simulink model "measurements"  (Simulink 8.5)
settings: Solver=ode45  StartTime=0.0  StopTime=10.0  RelTol=1e-3
libraries: powerlib x18
settings Model: Creator=Dr. Lotfifard  LastModifiedBy=PC  ExtModeTrigMode=oneshot  ExtModeArmWhenConnect=off
settings DataIOCC: LimitDataPoints=off
settings OptimizationCC: BlockReduction=off  BooleanDataType=off
settings DebuggingCC: SaveWithParameterizedLinksMsg=none  SignalResolutionControl=TryResolveAllWithWarning  MultiTaskDSMMsg=warning  MultiTaskCondExecSysMsg=none  FcnCallInpInsideContextMsg=UseLocalSettings  StrictBusMsg=None
settings HardwareCC: TargetUnknown=on

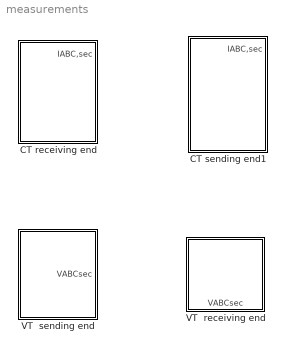
== system measurements ==
  CT receiving end : Subsystem  mask{TC=1.2}
      mask prompts: TC "Maximum Normal Current"
  CT sending end1 : Subsystem  mask{TC=1.2}
      mask prompts: TC "Maximum Normal Current"
  VT  receiving end : Subsystem  mask{TP=1000}
      mask prompts: TP "Nominal Voltage,rms"
  VT  sending end : Subsystem  mask{TP=1000}
      mask prompts: TP "Nominal Voltage,rms"

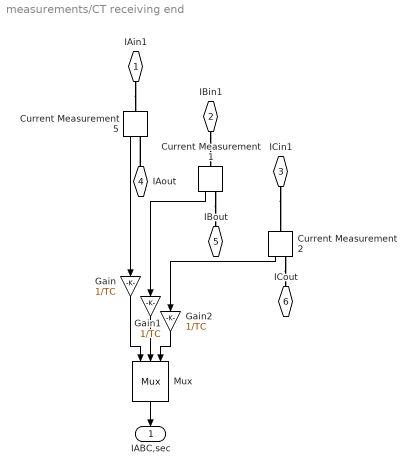
== system measurements/CT receiving end ==
  Current Measurement1 : powerlib/Measurements/Current Measurement  PhasorSimulation=off  OutputType=Complex  PSBequivalent=0
  Current Measurement2 : powerlib/Measurements/Current Measurement  PhasorSimulation=off  OutputType=Complex  PSBequivalent=0
  Current Measurement5 : powerlib/Measurements/Current Measurement  PhasorSimulation=off  OutputType=Complex  PSBequivalent=0
  Gain : Gain  Gain=1/TC  SaturateOnIntegerOverflow=on  OutDataTypeStr=Inherit: Same as input  ParamDataTypeStr=Inherit: Same as input
  Gain1 : Gain  Gain=1/TC  SaturateOnIntegerOverflow=on  OutDataTypeStr=Inherit: Same as input  ParamDataTypeStr=Inherit: Same as input
  Gain2 : Gain  Gain=1/TC  SaturateOnIntegerOverflow=on  OutDataTypeStr=Inherit: Same as input  ParamDataTypeStr=Inherit: Same as input
  Mux : Mux  Inputs=3
  IAin1 : PMIOPort  Port=1  Side=Left
  IBin1 : PMIOPort  Port=2  Side=Left
  ICin1 : PMIOPort  Port=3  Side=Left
  IAout : PMIOPort  Port=4  Side=Right
  IBout : PMIOPort  Port=5  Side=Right
  ICout : PMIOPort  Port=6  Side=Right
  IABC,sec : Outport  InitialOutput=0
  wires:
  Mux/1 -> IABC,sec/1
  Current Measurement2/1 -> Gain2/1
  Gain/1 -> Mux/1
  Gain1/1 -> Mux/2
  Gain2/1 -> Mux/3
  Current Measurement1/1 -> Gain1/1
  Current Measurement5/1 -> Gain/1
  connections:
  IAin1/RConn1 -- Current Measurement5/LConn1
  ICin1/RConn1 -- Current Measurement2/LConn1
  IBin1/RConn1 -- Current Measurement1/LConn1
  IAout/RConn1 -- Current Measurement5/RConn1
  Current Measurement1/RConn1 -- IBout/RConn1
  Current Measurement2/RConn1 -- ICout/RConn1

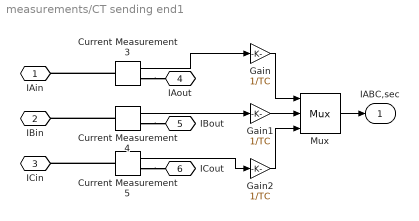
== system measurements/CT sending end1 ==
  Current Measurement3 : powerlib/Measurements/Current Measurement  PhasorSimulation=off  OutputType=Complex  PSBequivalent=0
  Current Measurement4 : powerlib/Measurements/Current Measurement  PhasorSimulation=off  OutputType=Complex  PSBequivalent=0
  Current Measurement5 : powerlib/Measurements/Current Measurement  PhasorSimulation=off  OutputType=Complex  PSBequivalent=0
  Gain : Gain  Gain=1/TC  SaturateOnIntegerOverflow=on  OutDataTypeStr=Inherit: Same as input  ParamDataTypeStr=Inherit: Same as input
  Gain1 : Gain  Gain=1/TC  SaturateOnIntegerOverflow=on  OutDataTypeStr=Inherit: Same as input  ParamDataTypeStr=Inherit: Same as input
  Gain2 : Gain  Gain=1/TC  SaturateOnIntegerOverflow=on  OutDataTypeStr=Inherit: Same as input  ParamDataTypeStr=Inherit: Same as input
  Mux : Mux  Inputs=3
  IAin : PMIOPort  Port=1  Side=Left
  IBin : PMIOPort  Port=2  Side=Left
  ICin : PMIOPort  Port=3  Side=Left
  IAout : PMIOPort  Port=4  Side=Right
  IBout : PMIOPort  Port=5  Side=Right
  ICout : PMIOPort  Port=6  Side=Right
  IABC,sec : Outport  InitialOutput=0
  wires:
  Mux/1 -> IABC,sec/1
  Gain/1 -> Mux/1
  Gain1/1 -> Mux/2
  Gain2/1 -> Mux/3
  Current Measurement3/1 -> Gain/1
  Current Measurement4/1 -> Gain1/1
  Current Measurement5/1 -> Gain2/1
  connections:
  Current Measurement4/RConn1 -- IBout/RConn1
  Current Measurement3/LConn1 -- IAin/RConn1
  Current Measurement4/LConn1 -- IBin/RConn1
  Current Measurement3/RConn1 -- IAout/RConn1
  Current Measurement5/LConn1 -- ICin/RConn1
  Current Measurement5/RConn1 -- ICout/RConn1

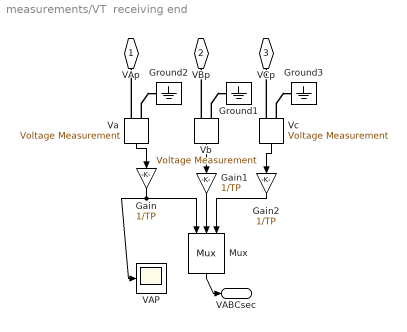
== system measurements/VT  receiving end ==
  Gain : Gain  Gain=1/TP  SaturateOnIntegerOverflow=on  OutDataTypeStr=Inherit: Same as input  ParamDataTypeStr=Inherit: Same as input
  Gain1 : Gain  Gain=1/TP  SaturateOnIntegerOverflow=on  OutDataTypeStr=Inherit: Same as input  ParamDataTypeStr=Inherit: Same as input
  Gain2 : Gain  Gain=1/TP  SaturateOnIntegerOverflow=on  OutDataTypeStr=Inherit: Same as input  ParamDataTypeStr=Inherit: Same as input
  Ground1 : powerlib/Elements/Ground  LConnTagsString=a
  Ground2 : powerlib/Elements/Ground  LConnTagsString=a
  Ground3 : powerlib/Elements/Ground  LConnTagsString=a
  Mux : Mux  Inputs=3
  VAP : Scope
      settings: TickLabels=on  YMin=-1.5  YMax=1.75
  Va : powerlib/Measurements/Voltage Measurement  PhasorSimulation=off  OutputType=Complex  PSBequivalent=0
  Vb : powerlib/Measurements/Voltage Measurement  PhasorSimulation=off  OutputType=Complex  PSBequivalent=0
  Vc : powerlib/Measurements/Voltage Measurement  PhasorSimulation=off  OutputType=Complex  PSBequivalent=0
  VAp : PMIOPort  Port=1  Side=Left
  VBp : PMIOPort  Port=2  Side=Left
  VCp : PMIOPort  Port=3  Side=Left
  VABCsec : Outport
  wires:
  Gain/1 -> VAP/1, Mux/1
  Mux/1 -> VABCsec/1
  Gain2/1 -> Mux/3
  Gain1/1 -> Mux/2
  Vb/1 -> Gain1/1
  Vc/1 -> Gain2/1
  Va/1 -> Gain/1
  connections:
  Va/LConn1 -- VAp/RConn1
  Va/LConn2 -- Ground2/LConn1
  Vb/LConn1 -- VBp/RConn1
  Vb/LConn2 -- Ground1/LConn1
  Vc/LConn1 -- VCp/RConn1
  Vc/LConn2 -- Ground3/LConn1

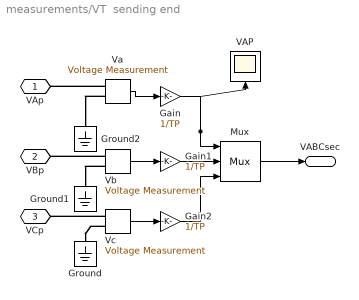
== system measurements/VT  sending end ==
  Gain : Gain  Gain=1/TP  SaturateOnIntegerOverflow=on  OutDataTypeStr=Inherit: Same as input  ParamDataTypeStr=Inherit: Same as input
  Gain1 : Gain  Gain=1/TP  SaturateOnIntegerOverflow=on  OutDataTypeStr=Inherit: Same as input  ParamDataTypeStr=Inherit: Same as input
  Gain2 : Gain  Gain=1/TP  SaturateOnIntegerOverflow=on  OutDataTypeStr=Inherit: Same as input  ParamDataTypeStr=Inherit: Same as input
  Ground : powerlib/Elements/Ground  LConnTagsString=a
  Ground1 : powerlib/Elements/Ground  LConnTagsString=a
  Ground2 : powerlib/Elements/Ground  LConnTagsString=a
  Mux : Mux  Inputs=3
  VAP : Scope
      settings: TickLabels=on  YMin=-1.5  YMax=1.75
  Va : powerlib/Measurements/Voltage Measurement  PhasorSimulation=off  OutputType=Complex  PSBequivalent=0
  Vb : powerlib/Measurements/Voltage Measurement  PhasorSimulation=off  OutputType=Complex  PSBequivalent=0
  Vc : powerlib/Measurements/Voltage Measurement  PhasorSimulation=off  OutputType=Complex  PSBequivalent=0
  VAp : PMIOPort  Port=1  Side=Left
  VBp : PMIOPort  Port=2  Side=Left
  VCp : PMIOPort  Port=3  Side=Left
  VABCsec : Outport
  wires:
  Gain1/1 -> Mux/2
  Vb/1 -> Gain1/1
  Mux/1 -> VABCsec/1
  Gain2/1 -> Mux/3
  Vc/1 -> Gain2/1
  Va/1 -> Gain/1
  Gain/1 -> Mux/1, VAP/1
  connections:
  Vc/LConn2 -- Ground/LConn1
  Vb/LConn2 -- Ground1/LConn1
  Va/LConn2 -- Ground2/LConn1
  Va/LConn1 -- VAp/RConn1
  Vb/LConn1 -- VBp/RConn1
  Vc/LConn1 -- VCp/RConn1
